simulink library "func_block_library"  (R2017b)
settings: Solver=VariableStepAuto  StartTime=0.0  StopTime=10.0  RelTol=1e-3
settings Model: Creator=81068  LastModifiedBy=81068

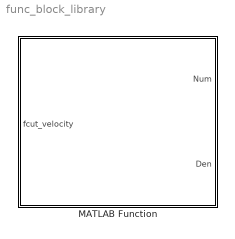
== system func_block_library ==
  MATLAB Function : MATLAB Function  TreatAsAtomicUnit=on

== matlab function func_block_library/MATLAB Function ==
  data: fcut_velocity input; Num output; Den output
function [Num, Den] = velocity_filter_param(fcut_velocity)
sample_time = 1/2000;
lpf_damping = sqrt(2)/2; % Butterworth filter damping
B1_lpf_velocity = -2*exp(-lpf_damping*fcut_velocity*sample_time)*cos(fcut_velocity*sample_time*sqrt(1-lpf_damping^2));
B2_lpf_velocity = exp(-2*lpf_damping*fcut_velocity*sample_time);
A_lpf_velocity = 1 + B1_lpf_velocity + B2_lpf_velocity;

Num = [ A_lpf_velocity 0 0];
Den = [ 1 B1_lpf_velocity B2_lpf_velocity];
end
